simulink model "TempCtrlClosedLoop"  (R2026a)
settings: Solver=ode3  StopTime=200  FixedStep=0.005
PreLoadFcn:
  | TempCtrlParameters();
values from neighbouring files (symbols this model uses):
  SetpointDefault = 37    [TempCtrlParameters.m]
settings Model: Creator=MatthiasJ  LastModifiedBy=Admin
settings DataIOCC: SignalLoggingSaveFormat=ModelDataLogs
settings OptimizationCC: LocalBlockOutputs=off
settings DebuggingCC: UnderspecifiedInitializationDetection=Classic
settings HardwareCC: ProdHWDeviceType=32-bit Generic
settings SFSimCC: SimTargetLang=C++
settings RTWCC: GenCodeOnly=on  GenerateReport=on  RTWVerbose=off  RetainRTWFile=on  TargetLang=C++
settings CodeAppCC: MaxIdLength=50.0
settings GRTTargetCC: CodeInterfacePackaging=C++ class  SubcomponentCodeInterfacePackaging=C++ class

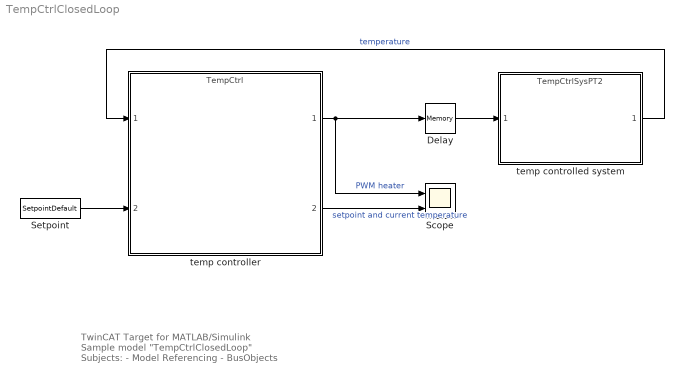
== system TempCtrlClosedLoop ==
  note: TwinCAT Target for MATLAB/Simulink
      | Sample model "TempCtrlClosedLoop"
      | Subjects:
      | - Model Referencing
      | - BusObjects
  Delay : Memory
  Scope : Scope  NumInputPorts=2
      settings: ActiveDisplayYMinimum=0.8986573475537738  ActiveDisplayYMaximum=1.1349089636018803
  Setpoint : Constant  Value=SetpointDefault
  temp controlled system : ModelReference  ModelNameDialog=TempCtrlSysPT2  ModelReferenceVersion=17.7
  temp controller : ModelReference  ModelNameDialog=TempCtrl  ModelReferenceVersion=17.19
  wires:
  temp controlled system/1 -> temp controller/1  "temperature"
  Delay/1 -> temp controlled system/1
  temp controller/1 -> Delay/1, Scope/1  "PWM heater"
  temp controller/2 -> Scope/2  "setpoint and current temperature"
  Setpoint/1 -> temp controller/2
